simulink model "vehicle"  (R2022b)
settings: Solver=VariableStepAuto  StartTime=0.0  StopTime=10.0  RelTol=1e-3
model workspace: external: MATLAB File C:\Users\alexa\MATLAB\Projects\Sleipner\data\vehicle_data.m (data not in the file)
undefined symbols (not defined in the file): AeroDragCoeff, airDensity, frontArea, gravity, inclineAngle, magnitude, massVeh, rollingResistCoeff, signal1, signal2, signal3, signal4, signal5, signal7, Velocity
settings Model: Creator=alexa  LastModifiedBy=alexa

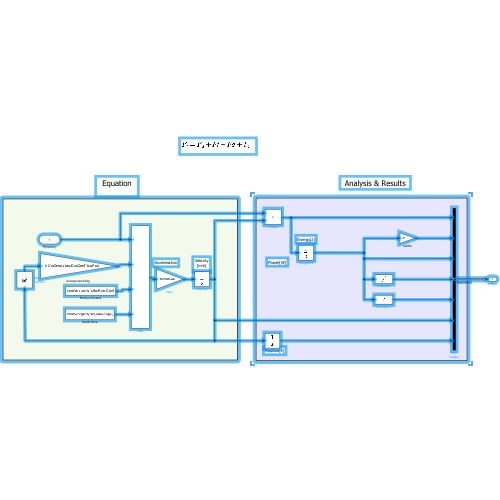
[thumbnail: Simulink's stored preview of the top-level diagram]
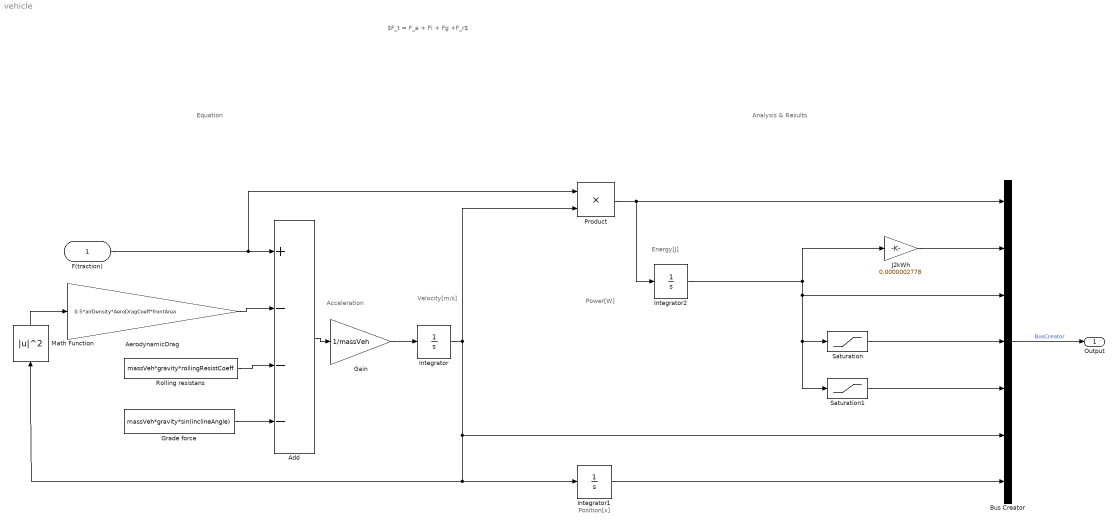
== system vehicle ==
  note: Equation
  note: Energy[J]
  note: Power[W]
  note: Acceleration
  note: Position[x]
  note: Velocity[m/s]
  note: $F_t = F_a + Fi + Fg +F_r$
  note: Analysis & Results
  F(traction) : Inport
  Add : Sum  Inputs=+---
  AerodynamicDrag : Gain  Gain=0.5*airDensity*AeroDragCoeff*frontArea
  Bus Creator : BusCreator  Inputs=signal1,signal2,signal3,signal4,signal5,Velocity,signal7  OutDataTypeStr=Bus: BusObject
  Gain : Gain  Gain=1/massVeh
  Grade force : Constant  Value=massVeh*gravity*sin(inclineAngle)
  Integrator : Integrator
  Integrator1 : Integrator
  Integrator2 : Integrator
  J2kWh : Gain  Gain=0.0000002778
  Math Function : Math  Operator=magnitude^2
  Product : Product
  Rolling resistans : Constant  Value=massVeh*gravity*rollingResistCoeff
  Saturation : Saturate  UpperLimit=inf  LowerLimit=0
  Saturation1 : Saturate  UpperLimit=0  LowerLimit=-inf
  Output : Outport
  wires:
  AerodynamicDrag/1 -> Add/2
  Math Function/1 -> AerodynamicDrag/1
  Add/1 -> Gain/1
  F(traction)/1 -> Product/1, Add/1
  Rolling resistans/1 -> Add/3
  Grade force/1 -> Add/4
  Gain/1 -> Integrator/1
  Integrator1/1 -> Bus Creator/7
  Integrator/1 -> Product/2, Bus Creator/6, Integrator1/1, Math Function/1
  Product/1 -> Bus Creator/1, Integrator2/1
  Integrator2/1 -> J2kWh/1, Saturation1/1, Saturation/1, Bus Creator/3
  J2kWh/1 -> Bus Creator/2
  Saturation/1 -> Bus Creator/4
  Saturation1/1 -> Bus Creator/5
  Bus Creator/1 -> Output/1  "BusCreator"
